simulink model "me132LabPartG"  (R2021a)
settings: Solver=VariableStepAuto  StartTime=0.0  StopTime=10.0  RelTol=1e-3
undefined symbols (not defined in the file): alpha, beta, Kfb, Kff
settings Model: Creator=kaiyu  LastModifiedBy=kaiyu

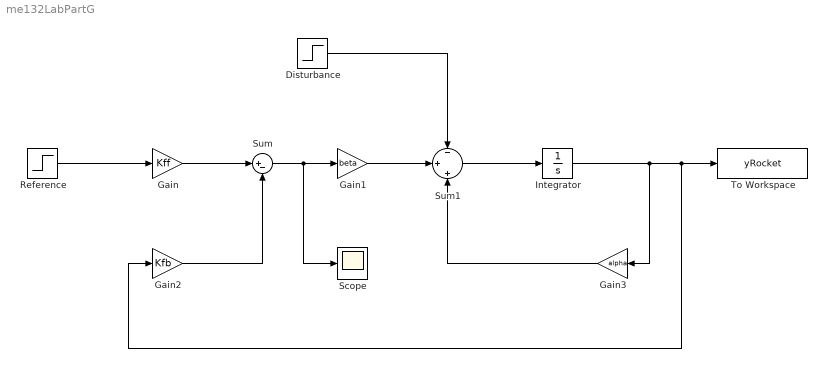
== system me132LabPartG ==
  Disturbance : Step  Time=6  SampleTime=0
  Gain : Gain  Gain=Kff
  Gain1 : Gain  Gain=beta
  Gain2 : Gain  Gain=Kfb
  Gain3 : Gain  Gain=alpha
  Integrator : Integrator
  Reference : Step  SampleTime=0
  Scope : Scope
  Sum : Sum  Inputs=|+-
  Sum1 : Sum  Inputs=-|+|+
  To Workspace : ToWorkspace  VariableName=yRocket  SaveFormat=Structure With Time  SampleTime=-1
  wires:
  Gain3/1 -> Sum1/3
  Integrator/1 -> Gain3/1, Gain2/1, To Workspace/1
  Sum1/1 -> Integrator/1
  Gain1/1 -> Sum1/2
  Sum/1 -> Scope/1, Gain1/1
  Gain/1 -> Sum/1
  Reference/1 -> Gain/1
  Gain2/1 -> Sum/2
  Disturbance/1 -> Sum1/1
